simulink model "OMAP"  (R2018b)
settings: Solver=FixedStepDiscrete  StartTime=0.0  StopTime=10.0  FixedStep=0.01  RelTol=1e-3
values from neighbouring files (symbols this model uses):
  Clb_ICADirect_LaneDisp_StateFive = Simulink.Parameter    [omap_ver_442.m]
  Clb_ICADirect_LaneDisp_StateFour = Simulink.Parameter    [omap_ver_442.m]
  Clb_ICADirect_LaneDisp_StateOne = Simulink.Parameter    [omap_ver_442.m]
  Clb_ICADirect_LaneDisp_StateThree = Simulink.Parameter    [omap_ver_442.m]
  Clb_ICADirect_LaneDisp_StateTwo = Simulink.Parameter    [omap_ver_442.m]
  Clb_ICADirect_LaneDisp_StateZero = Simulink.Parameter    [omap_ver_442.m]
  Clb_ICADirect_LaneDispSW = Simulink.Parameter    [omap_ver_442.m]
  Clb_ICADirect_TrnLghtsCom_Switch = Simulink.Parameter    [omap_ver_442.m]
  Clb_ICADirect_TrnLghtsCom_Value = Simulink.Parameter    [omap_ver_442.m]
  Clb_ICADirect_TrnLghtsCrtl_Inhb = Simulink.Parameter    [omap_ver_442.m]
  OMAP_ACCAEB_EMSESC_Decel = Simulink.Parameter    [omap_ver_442.m]
  OMAP_ACCFCW_IC_Decel = Simulink.Parameter    [omap_ver_442.m]
  OMAP_clb_ACC_RVVReqType = Simulink.Parameter    [omap_ver_442.m]
  OMAP_clb_ACC_RVVReqType_Switch = Simulink.Parameter    [omap_ver_442.m]
  OMAP_clb_ACCHeadwayDisplay = Simulink.Parameter    [omap_ver_442.m]
  OMAP_clb_ACCHeadwayDisplay_Switch = Simulink.Parameter    [omap_ver_442.m]
  OMAP_clb_ACCHeadwayIcon = Simulink.Parameter    [omap_ver_442.m]
  OMAP_clb_ACCHeadwayIcon_Switch = Simulink.Parameter    [omap_ver_442.m]
  OMAP_clb_ACCMessagePrompt = Simulink.Parameter    [omap_ver_442.m]
  OMAP_clb_ACCMessagePrompt_Switch = Simulink.Parameter    [omap_ver_442.m]
  OMAP_clb_ACCRequestEPB = Simulink.Parameter    [omap_ver_442.m]
  OMAP_clb_ACCRequestEPB_Switch = Simulink.Parameter    [omap_ver_442.m]
  OMAP_clb_ACCSetSpeed = Simulink.Parameter    [omap_ver_442.m]
  OMAP_clb_ACCSetSpeed_Switch = Simulink.Parameter    [omap_ver_442.m]
  OMAP_clb_ACCSetSpeedDis = Simulink.Parameter    [omap_ver_442.m]
  OMAP_clb_ACCSetSpeedDis_Switch = Simulink.Parameter    [omap_ver_442.m]
  OMAP_clb_ACCState = Simulink.Parameter    [omap_ver_442.m]
  OMAP_clb_ACCState_Switch = Simulink.Parameter    [omap_ver_442.m]
  OMAP_clb_ACCStatusIconDis = Simulink.Parameter    [omap_ver_442.m]
  OMAP_clb_ACCStatusIconDis_Switch = Simulink.Parameter    [omap_ver_442.m]
  OMAP_clb_ACCTorqueReq = Simulink.Parameter    [omap_ver_442.m]
  OMAP_clb_ACCTorqueReq_Switch = Simulink.Parameter    [omap_ver_442.m]
  OMAP_clb_ADAS_State = Simulink.Parameter    [omap_ver_442.m]
  OMAP_clb_ADAS_State_Switch = Simulink.Parameter    [omap_ver_442.m]
  OMAP_clb_AEBAlertReq = Simulink.Parameter    [omap_ver_442.m]
  OMAP_clb_AEBAlertReq_Switch = Simulink.Parameter    [omap_ver_442.m]
  OMAP_clb_AEBBrakingProg = Simulink.Parameter    [omap_ver_442.m]
  OMAP_clb_AEBBrakingProg_Switch = Simulink.Parameter    [omap_ver_442.m]
  OMAP_clb_AEBFaultStatus = Simulink.Parameter    [omap_ver_442.m]
  OMAP_clb_AEBFaultStatus_Switch = Simulink.Parameter    [omap_ver_442.m]
  OMAP_clb_AEBMassageDisp = Simulink.Parameter    [omap_ver_442.m]
  OMAP_clb_AEBMassageDisp_Switch = Simulink.Parameter    [omap_ver_442.m]
  OMAP_clb_AEBState = Simulink.Parameter    [omap_ver_442.m]
  OMAP_clb_AEBState_Switch = Simulink.Parameter    [omap_ver_442.m]
  OMAP_clb_AEBSwitchStatus = Simulink.Parameter    [omap_ver_442.m]
  OMAP_clb_AEBSwitchStatus_Switch = Simulink.Parameter    [omap_ver_442.m]
  OMAP_clb_BrakeRequest = Simulink.Parameter    [omap_ver_442.m]
  OMAP_clb_BrakeRequest_Switch = Simulink.Parameter    [omap_ver_442.m]
  OMAP_clb_DecelerationSet = Simulink.Parameter    [omap_ver_442.m]
  OMAP_clb_DecelerationSet_Switch = Simulink.Parameter    [omap_ver_442.m]
  OMAP_clb_DecelerationType = Simulink.Parameter    [omap_ver_442.m]
  OMAP_clb_DecelerationType_Switch = Simulink.Parameter    [omap_ver_442.m]
  OMAP_clb_DeclControlReq = Simulink.Parameter    [omap_ver_442.m]
  OMAP_clb_DeclControlReq_Switch = Simulink.Parameter    [omap_ver_442.m]
  OMAP_clb_DownorUpGearMinTime = Simulink.Parameter    [omap_ver_442.m]
  OMAP_clb_DownorUpGearMinTime_Switch = Simulink.Parameter    [omap_ver_442.m]
  OMAP_clb_ELKPopupMessage = Simulink.Parameter    [omap_ver_442.m]
  OMAP_clb_ELKPopupMessage_Switch = Simulink.Parameter    [omap_ver_442.m]
  OMAP_clb_ELKSts = Simulink.Parameter    [omap_ver_442.m]
  OMAP_clb_ELKSts_Switch = Simulink.Parameter    [omap_ver_442.m]
  OMAP_clb_ESAFaultSt = Simulink.Parameter    [omap_ver_442.m]
  OMAP_clb_ESAFaultSt_Switch = Simulink.Parameter    [omap_ver_442.m]
  OMAP_clb_ESARequest = Simulink.Parameter    [omap_ver_442.m]
  OMAP_clb_ESARequest_Switch = Simulink.Parameter    [omap_ver_442.m]
  OMAP_clb_ESAState = Simulink.Parameter    [omap_ver_442.m]
  OMAP_clb_ESAState_Switch = Simulink.Parameter    [omap_ver_442.m]
  OMAP_clb_ESATorqueReq = Simulink.Parameter    [omap_ver_442.m]
  OMAP_clb_ESATorqueReq_Switch = Simulink.Parameter    [omap_ver_442.m]
  OMAP_clb_ESCDriveOff = Simulink.Parameter    [omap_ver_442.m]
  OMAP_clb_ESCDriveOff_Switch = Simulink.Parameter    [omap_ver_442.m]
  OMAP_clb_ESCHoldReq = Simulink.Parameter    [omap_ver_442.m]
  OMAP_clb_ESCHoldReq_Switch = Simulink.Parameter    [omap_ver_442.m]
  OMAP_clb_Handsoffwarning = Simulink.Parameter    [omap_ver_442.m]
  OMAP_clb_Handsoffwarning_Switch = Simulink.Parameter    [omap_ver_442.m]
  OMAP_clb_HapticAlarmReq = Simulink.Parameter    [omap_ver_442.m]
  OMAP_clb_HapticAlarmReq_Switch = Simulink.Parameter    [omap_ver_442.m]
  OMAP_clb_HMIPopupMassage = Simulink.Parameter    [omap_ver_442.m]
  OMAP_clb_HMIPopupMassage_Switch = Simulink.Parameter    [omap_ver_442.m]
  OMAP_clb_HWAActionSts = Simulink.Parameter    [omap_ver_442.m]
  OMAP_clb_HWAActionSts_Switch = Simulink.Parameter    [omap_ver_442.m]
  OMAP_clb_HWAMode = Simulink.Parameter    [omap_ver_442.m]
  OMAP_clb_HWAMode_Switch = Simulink.Parameter    [omap_ver_442.m]
  OMAP_clb_HWATurnOnIdctr = Simulink.Parameter    [omap_ver_442.m]
  OMAP_clb_HWATurnOnIdctr_Switch = Simulink.Parameter    [omap_ver_442.m]
  OMAP_clb_ICAMassageDisp = Simulink.Parameter    [omap_ver_442.m]
  OMAP_clb_ICAMassageDisp_Switch = Simulink.Parameter    [omap_ver_442.m]
  OMAP_clb_ICAStatusIcon = Simulink.Parameter    [omap_ver_442.m]
  OMAP_clb_ICAStatusIcon_Switch = Simulink.Parameter    [omap_ver_442.m]
  OMAP_clb_ISLCDriverRemind = Simulink.Parameter    [omap_ver_442.m]
  OMAP_clb_ISLCDriverRemind_Switch = Simulink.Parameter    [omap_ver_442.m]
  OMAP_clb_ISLCState = Simulink.Parameter    [omap_ver_442.m]
  OMAP_clb_ISLCState_Switch = Simulink.Parameter    [omap_ver_442.m]
  OMAP_clb_JAFaultSt = Simulink.Parameter    [omap_ver_442.m]
  OMAP_clb_JAFaultSt_Switch = Simulink.Parameter    [omap_ver_442.m]
  OMAP_clb_LCAPopupMessage = Simulink.Parameter    [omap_ver_442.m]
  OMAP_clb_LCAPopupMessage_Switch = Simulink.Parameter    [omap_ver_442.m]
  OMAP_clb_LCAStatusDisplay = Simulink.Parameter    [omap_ver_442.m]
  OMAP_clb_LCAStatusDisplay_Switch = Simulink.Parameter    [omap_ver_442.m]
  OMAP_clb_LDWStatusDisplay = Simulink.Parameter    [omap_ver_442.m]
  OMAP_clb_LDWStatusDisplay_Switch = Simulink.Parameter    [omap_ver_442.m]
  OMAP_clb_LDWWarningSt = Simulink.Parameter    [omap_ver_442.m]
  OMAP_clb_LDWWarningSt_Switch = Simulink.Parameter    [omap_ver_442.m]
  OMAP_clb_LightControlValid = Simulink.Parameter    [omap_ver_442.m]
  OMAP_clb_LightControlValid_Switch = Simulink.Parameter    [omap_ver_442.m]
  OMAP_clb_LKAActivation = Simulink.Parameter    [omap_ver_442.m]
  OMAP_clb_LKAActivation_Switch = Simulink.Parameter    [omap_ver_442.m]
  OMAP_clb_LKAAngleReq = Simulink.Parameter    [omap_ver_442.m]
  OMAP_clb_LKAAngleReq_Switch = Simulink.Parameter    [omap_ver_442.m]
  OMAP_clb_LKAMode = Simulink.Parameter    [omap_ver_442.m]
  OMAP_clb_LKAMode_Switch = Simulink.Parameter    [omap_ver_442.m]
  OMAP_clb_LKAorELK_CoolTime = Simulink.Parameter    [omap_ver_442.m]
  OMAP_clb_LKAState = Simulink.Parameter    [omap_ver_442.m]
  OMAP_clb_LKAState_Switch = Simulink.Parameter    [omap_ver_442.m]
  OMAP_clb_LKAStatusDisplay = Simulink.Parameter    [omap_ver_442.m]
  OMAP_clb_LKAStatusDisplay_Switch = Simulink.Parameter    [omap_ver_442.m]
  OMAP_clb_LKASwitchState = Simulink.Parameter    [omap_ver_442.m]
  OMAP_clb_LKASwitchState_Switch = Simulink.Parameter    [omap_ver_442.m]
  OMAP_clb_LKATorqFactReq = Simulink.Parameter    [omap_ver_442.m]
  OMAP_clb_LKATorqFactReq_Switch = Simulink.Parameter    [omap_ver_442.m]
  OMAP_clb_PrefillRequest = Simulink.Parameter    [omap_ver_442.m]
  ... (+36 more)
libraries: simulink x184, canmsglib x2
(part 7 of 14)

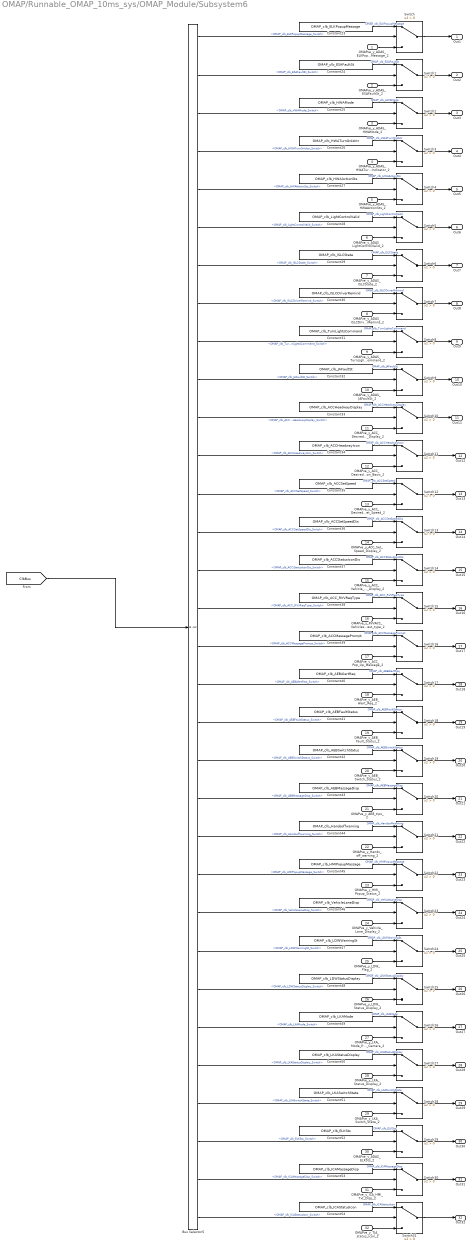
== system OMAP/Runnable_OMAP_10ms_sys/OMAP_Module/Subsystem6 ==
  OMAPve_y_ADAS_ELKPopupMessage_2 : Inport
  OMAPve_y_ADAS_ESAFaultSt_2 : Inport  Port=2
  OMAPve_y_ADAS_HWAMode_2 : Inport  Port=3
  OMAPve_y_ADAS_HWATurnOnIndicator_2 : Inport  Port=4
  OMAPve_y_ADAS_HWAActionSts_2 : Inport  Port=5
  OMAPve_y_ADAS_LightControlValid_2 : Inport  Port=6
  OMAPve_y_ADAS_ISLCState_2 : Inport  Port=7
  OMAPve_y_ADAS_ISLCDriverRemind_2 : Inport  Port=8
  OMAPve_y_ADAS_TurnLightsCommand_2 : Inport  Port=9
  OMAPve_y_ADAS_JAFaultSt_2 : Inport  Port=10
  OMAPve_y_ACC_DesiredHeadway_Display_2 : Inport  Port=11
  OMAPve_y_ACC_DesiredHeadway_Icon_Basic_2 : Inport  Port=12
  OMAPve_y_ACC_Desired_Set_Speed_2 : Inport  Port=13
  OMAPve_y_ACC_Set_Speed_Display_2 : Inport  Port=14
  OMAPve_y_ACC_Vehicle_Icon_Display_2 : Inport  Port=15
  OMAPve_y_RVVACC_Vehiclespeed_request_type_2 : Inport  Port=16
  OMAPve_y_ACC_Pop_Up_Message_2 : Inport  Port=17
  OMAPve_y_AEB_Alert_Req_2 : Inport  Port=18
  OMAPve_y_AEB_Fault_Status_2 : Inport  Port=19
  OMAPve_y_AEB_Switch_Status_2 : Inport  Port=20
  OMAPve_y_AEB_tips_2 : Inport  Port=21
  OMAPve_y_Hands_off_warning_2 : Inport  Port=22
  OMAPve_y_HMI_Popup_Status_2 : Inport  Port=23
  OMAPve_y_Vehicle_Lane_Display_2 : Inport  Port=24
  OMAPve_y_LDW_Flag_2 : Inport  Port=25
  OMAPve_y_LDW_Status_Display_2 : Inport  Port=26
  OMAPve_y_LKA_Mode_from_Camera_2 : Inport  Port=27
  OMAPve_y_LKA_Status_Display_2 : Inport  Port=28
  OMAPve_y_LKA_Switch_State_2 : Inport  Port=29
  OMAPve_y_ADAS_ELKSts_2 : Inport  Port=30
  OMAPve_y_ICA_HMI_Txt_Disp_2 : Inport  Port=31
  OMAPve_y_TJA_status_icon_2 : Inport  Port=32
  Bus Selector5 : BusSelector  OutputSignals=OMAP_clb_ELKPopupMessage_Switch,OMAP_clb_ESAFaultSt_Switch,OMAP_clb_HWAMode_Switch,OMAP_clb_HWATurnOnIdctr_Switch,OMAP_clb_HWAActionSts_Switch,OMAP_clb_LightControlValid_Switch,OMAP_clb_ISLCState_Switch,OMAP_clb_ISLCDriverRemind_Switch,OMAP_clb_TurnLightsCommand_Switch,OMAP_clb_JAFaultSt_Switch,OMAP_clb_ACCHeadwayDisplay_Switch,OMAP_clb_ACCHeadwayIcon_Switch,OMAP_clb_ACCSetSpeed_Switch,OMAP_clb_ACCSetSpeedDis_Switch,OMAP_clb_ACCStatusIconDis_Switch,OMAP_clb_ACC_RVVReqType_Switch,OMAP_clb_ACCMessagePrompt_Switch,OMAP_clb_AEBAlertReq_Switch,OMAP_clb_AEBFaultStatus_Switch,OMAP_clb_AEBSwitchStatus_Switch,OMAP_clb_AEBMassageDisp_Switch,OMAP_clb_Handsoffwarning_Switch,OMAP_clb_HMIPopupMassage_Switch,OMAP_clb_VehicleLaneDisp_Switch,OMAP_clb_LDWWarningSt_Switch,OMAP_clb_LDWStatusDisplay_Switch,OMAP_clb_LKAMode_Switch,OMAP_clb_LKAStatusDisplay_Switch,OMAP_clb_LKASwitchState_Switch,OMAP_clb_ELKSts_Switch,OMAP_clb_ICAMassageDisp_Switch,OMAP_clb_ICAStatusIcon_Switch
  Constant23 : Constant  Value=OMAP_clb_ELKPopupMessage
  Constant24 : Constant  Value=OMAP_clb_ESAFaultSt
  Constant25 : Constant  Value=OMAP_clb_HWAMode
  Constant26 : Constant  Value=OMAP_clb_HWATurnOnIdctr
  Constant27 : Constant  Value=OMAP_clb_HWAActionSts
  Constant28 : Constant  Value=OMAP_clb_LightControlValid
  Constant29 : Constant  Value=OMAP_clb_ISLCState
  Constant30 : Constant  Value=OMAP_clb_ISLCDriverRemind
  Constant31 : Constant  Value=OMAP_clb_TurnLightsCommand
  Constant32 : Constant  Value=OMAP_clb_JAFaultSt
  Constant33 : Constant  Value=OMAP_clb_ACCHeadwayDisplay
  Constant34 : Constant  Value=OMAP_clb_ACCHeadwayIcon
  Constant35 : Constant  Value=OMAP_clb_ACCSetSpeed
  Constant36 : Constant  Value=OMAP_clb_ACCSetSpeedDis
  Constant37 : Constant  Value=OMAP_clb_ACCStatusIconDis
  Constant38 : Constant  Value=OMAP_clb_ACC_RVVReqType
  Constant39 : Constant  Value=OMAP_clb_ACCMessagePrompt
  Constant40 : Constant  Value=OMAP_clb_AEBAlertReq
  Constant41 : Constant  Value=OMAP_clb_AEBFaultStatus
  Constant42 : Constant  Value=OMAP_clb_AEBSwitchStatus
  Constant43 : Constant  Value=OMAP_clb_AEBMassageDisp
  Constant44 : Constant  Value=OMAP_clb_Handsoffwarning
  Constant45 : Constant  Value=OMAP_clb_HMIPopupMassage
  Constant46 : Constant  Value=OMAP_clb_VehicleLaneDisp
  Constant47 : Constant  Value=OMAP_clb_LDWWarningSt
  Constant48 : Constant  Value=OMAP_clb_LDWStatusDisplay
  Constant49 : Constant  Value=OMAP_clb_LKAMode
  Constant50 : Constant  Value=OMAP_clb_LKAStatusDisplay
  Constant51 : Constant  Value=OMAP_clb_LKASwitchState
  Constant52 : Constant  Value=OMAP_clb_ELKSts
  Constant53 : Constant  Value=OMAP_clb_ICAMassageDisp
  Constant54 : Constant  Value=OMAP_clb_ICAStatusIcon
  Switch{,1..31} (32 alike) : Switch  Criteria=u2 > Threshold
  Out1 : Outport
  Out2 : Outport  Port=2
  Out3 : Outport  Port=3
  Out4 : Outport  Port=4
  Out5 : Outport  Port=5
  Out6 : Outport  Port=6
  Out7 : Outport  Port=7
  Out8 : Outport  Port=8
  Out9 : Outport  Port=9
  Out10 : Outport  Port=10
  Out11 : Outport  Port=11
  Out12 : Outport  Port=12
  Out13 : Outport  Port=13
  Out14 : Outport  Port=14
  Out15 : Outport  Port=15
  Out16 : Outport  Port=16
  Out17 : Outport  Port=17
  Out18 : Outport  Port=18
  Out19 : Outport  Port=19
  Out20 : Outport  Port=20
  Out21 : Outport  Port=21
  Out22 : Outport  Port=22
  Out23 : Outport  Port=23
  Out24 : Outport  Port=24
  Out25 : Outport  Port=25
  Out26 : Outport  Port=26
  Out27 : Outport  Port=27
  Out28 : Outport  Port=28
  Out29 : Outport  Port=29
  Out30 : Outport  Port=30
  Out31 : Outport  Port=31
  Out32 : Outport  Port=32
  wires:
  Switch10/1 -> Out11/1
  OMAPve_y_ACC_DesiredHeadway_Display_2/1 -> Switch10/3
  Bus Selector5/11 -> Switch10/2  "<OMAP_clb_ACCHeadwayDisplay_Switch>"
  OMAPve_y_ADAS_JAFaultSt_2/1 -> Switch9/3
  Switch9/1 -> Out10/1
  Bus Selector5/10 -> Switch9/2  "<OMAP_clb_JAFaultSt_Switch>"
  OMAPve_y_ADAS_TurnLightsCommand_2/1 -> Switch8/3
  Bus Selector5/9 -> Switch8/2  "<OMAP_clb_TurnLightsCommand_Switch>"
  Switch8/1 -> Out9/1
  Switch7/1 -> Out8/1
  OMAPve_y_ADAS_ISLCDriverRemind_2/1 -> Switch7/3
  Bus Selector5/8 -> Switch7/2  "<OMAP_clb_ISLCDriverRemind_Switch>"
  Switch6/1 -> Out7/1
  OMAPve_y_ADAS_ISLCState_2/1 -> Switch6/3
  Bus Selector5/7 -> Switch6/2  "<OMAP_clb_ISLCState_Switch>"
  Switch5/1 -> Out6/1
  OMAPve_y_ADAS_LightControlValid_2/1 -> Switch5/3
  Bus Selector5/6 -> Switch5/2  "<OMAP_clb_LightControlValid_Switch>"
  Switch4/1 -> Out5/1
  Bus Selector5/5 -> Switch4/2  "<OMAP_clb_HWAActionSts_Switch>"
  OMAPve_y_ADAS_HWAActionSts_2/1 -> Switch4/3
  Bus Selector5/2 -> Switch1/2  "<OMAP_clb_ESAFaultSt_Switch>"
  Switch2/1 -> Out3/1
  OMAPve_y_ADAS_HWATurnOnIndicator_2/1 -> Switch3/3
  OMAPve_y_ADAS_HWAMode_2/1 -> Switch2/3
  OMAPve_y_ADAS_ESAFaultSt_2/1 -> Switch1/3
  Bus Selector5/1 -> Switch/2  "<OMAP_clb_ELKPopupMessage_Switch>"
  [ClbBus] -> Bus Selector5/1
  Bus Selector5/3 -> Switch2/2  "<OMAP_clb_HWAMode_Switch>"
  Bus Selector5/4 -> Switch3/2  "<OMAP_clb_HWATurnOnIdctr_Switch>"
  OMAPve_y_ADAS_ELKPopupMessage_2/1 -> Switch/3
  Switch1/1 -> Out2/1
  Switch3/1 -> Out4/1
  Switch/1 -> Out1/1
  Bus Selector5/12 -> Switch11/2  "<OMAP_clb_ACCHeadwayIcon_Switch>"
  OMAPve_y_ACC_DesiredHeadway_Icon_Basic_2/1 -> Switch11/3
  Switch11/1 -> Out12/1
  Bus Selector5/13 -> Switch12/2  "<OMAP_clb_ACCSetSpeed_Switch>"
  OMAPve_y_ACC_Desired_Set_Speed_2/1 -> Switch12/3
  Switch12/1 -> Out13/1
  Switch13/1 -> Out14/1
  OMAPve_y_ACC_Set_Speed_Display_2/1 -> Switch13/3
  Bus Selector5/14 -> Switch13/2  "<OMAP_clb_ACCSetSpeedDis_Switch>"
  Bus Selector5/15 -> Switch14/2  "<OMAP_clb_ACCStatusIconDis_Switch>"
  OMAPve_y_ACC_Vehicle_Icon_Display_2/1 -> Switch14/3
  Switch14/1 -> Out15/1
  Switch15/1 -> Out16/1
  OMAPve_y_RVVACC_Vehiclespeed_request_type_2/1 -> Switch15/3
  Bus Selector5/16 -> Switch15/2  "<OMAP_clb_ACC_RVVReqType_Switch>"
  Bus Selector5/17 -> Switch16/2  "<OMAP_clb_ACCMessagePrompt_Switch>"
  OMAPve_y_ACC_Pop_Up_Message_2/1 -> Switch16/3
  Switch16/1 -> Out17/1
  Switch17/1 -> Out18/1
  OMAPve_y_AEB_Alert_Req_2/1 -> Switch17/3
  Bus Selector5/18 -> Switch17/2  "<OMAP_clb_AEBAlertReq_Switch>"
  Bus Selector5/19 -> Switch18/2  "<OMAP_clb_AEBFaultStatus_Switch>"
  OMAPve_y_AEB_Fault_Status_2/1 -> Switch18/3
  Switch18/1 -> Out19/1
  Switch19/1 -> Out20/1
  OMAPve_y_AEB_Switch_Status_2/1 -> Switch19/3
  Bus Selector5/20 -> Switch19/2  "<OMAP_clb_AEBSwitchStatus_Switch>"
  Bus Selector5/21 -> Switch20/2  "<OMAP_clb_AEBMassageDisp_Switch>"
  OMAPve_y_AEB_tips_2/1 -> Switch20/3
  Switch20/1 -> Out21/1
  Switch21/1 -> Out22/1
  OMAPve_y_Hands_off_warning_2/1 -> Switch21/3
  Bus Selector5/22 -> Switch21/2  "<OMAP_clb_Handsoffwarning_Switch>"
  Bus Selector5/23 -> Switch22/2  "<OMAP_clb_HMIPopupMassage_Switch>"
  OMAPve_y_HMI_Popup_Status_2/1 -> Switch22/3
  Switch22/1 -> Out23/1
  Switch23/1 -> Out24/1
  OMAPve_y_Vehicle_Lane_Display_2/1 -> Switch23/3
  Bus Selector5/24 -> Switch23/2  "<OMAP_clb_VehicleLaneDisp_Switch>"
  Bus Selector5/25 -> Switch24/2  "<OMAP_clb_LDWWarningSt_Switch>"
  OMAPve_y_LDW_Flag_2/1 -> Switch24/3
  Switch24/1 -> Out25/1
  Switch25/1 -> Out26/1
  OMAPve_y_LDW_Status_Display_2/1 -> Switch25/3
  Bus Selector5/26 -> Switch25/2  "<OMAP_clb_LDWStatusDisplay_Switch>"
  Bus Selector5/27 -> Switch26/2  "<OMAP_clb_LKAMode_Switch>"
  OMAPve_y_LKA_Mode_from_Camera_2/1 -> Switch26/3
  Switch26/1 -> Out27/1
  Switch27/1 -> Out28/1
  OMAPve_y_LKA_Status_Display_2/1 -> Switch27/3
  Bus Selector5/28 -> Switch27/2  "<OMAP_clb_LKAStatusDisplay_Switch>"
  Bus Selector5/29 -> Switch28/2  "<OMAP_clb_LKASwitchState_Switch>"
  OMAPve_y_LKA_Switch_State_2/1 -> Switch28/3
  Switch28/1 -> Out29/1
  Switch29/1 -> Out30/1
  OMAPve_y_ADAS_ELKSts_2/1 -> Switch29/3
  Bus Selector5/30 -> Switch29/2  "<OMAP_clb_ELKSts_Switch>"
  Bus Selector5/31 -> Switch30/2  "<OMAP_clb_ICAMassageDisp_Switch>"
  OMAPve_y_ICA_HMI_Txt_Disp_2/1 -> Switch30/3
  Switch30/1 -> Out31/1
  Switch31/1 -> Out32/1
  OMAPve_y_TJA_status_icon_2/1 -> Switch31/3
  Bus Selector5/32 -> Switch31/2  "<OMAP_clb_ICAStatusIcon_Switch>"
  Constant23/1 -> Switch/1  "OMAP_clb_ELKPopupMessage"
  Constant24/1 -> Switch1/1  "OMAP_clb_ESAFaultSt"
  Constant25/1 -> Switch2/1  "OMAP_clb_HWAMode"
  Constant26/1 -> Switch3/1  "OMAP_clb_HWATurnOnIdctr"
  Constant27/1 -> Switch4/1  "OMAP_clb_HWAActionSts"
  Constant28/1 -> Switch5/1  "OMAP_clb_LightControlValid"
  Constant29/1 -> Switch6/1  "OMAP_clb_ISLCState"
  Constant30/1 -> Switch7/1  "OMAP_clb_ISLCDriverRemind"
  Constant31/1 -> Switch8/1  "OMAP_clb_TurnLightsCommand"
  Constant32/1 -> Switch9/1  "OMAP_clb_JAFaultSt"
  Constant33/1 -> Switch10/1  "OMAP_clb_ACCHeadwayDisplay"
  Constant34/1 -> Switch11/1  "OMAP_clb_ACCHeadwayIcon"
  Constant35/1 -> Switch12/1  "OMAP_clb_ACCSetSpeed"
  Constant36/1 -> Switch13/1  "OMAP_clb_ACCSetSpeedDis"
  Constant37/1 -> Switch14/1  "OMAP_clb_ACCStatusIconDis"
  Constant38/1 -> Switch15/1  "OMAP_clb_ACC_RVVReqType"
  Constant39/1 -> Switch16/1  "OMAP_clb_ACCMessagePrompt"
  Constant40/1 -> Switch17/1  "OMAP_clb_AEBAlertReq"
  Constant41/1 -> Switch18/1  "OMAP_clb_AEBFaultStatus"
  Constant42/1 -> Switch19/1  "OMAP_clb_AEBSwitchStatus"
  Constant43/1 -> Switch20/1  "OMAP_clb_AEBMassageDisp"
  Constant44/1 -> Switch21/1  "OMAP_clb_Handsoffwarning"
  Constant45/1 -> Switch22/1  "OMAP_clb_HMIPopupMassage"
  Constant46/1 -> Switch23/1  "OMAP_clb_VehicleLaneDisp"
  Constant47/1 -> Switch24/1  "OMAP_clb_LDWWarningSt"
  Constant48/1 -> Switch25/1  "OMAP_clb_LDWStatusDisplay"
  Constant49/1 -> Switch26/1  "OMAP_clb_LKAMode"
  Constant50/1 -> Switch27/1  "OMAP_clb_LKAStatusDisplay"
  Constant51/1 -> Switch28/1  "OMAP_clb_LKASwitchState"
  Constant52/1 -> Switch29/1  "OMAP_clb_ELKSts"
  Constant53/1 -> Switch30/1  "OMAP_clb_ICAMassageDisp"
  Constant54/1 -> Switch31/1  "OMAP_clb_ICAStatusIcon"

== system OMAP/Runnable_OMAP_10ms_sys/OMAP_Module/Subsystem7 ==
  OMAPve_y_ADAS_LCAStatusDisplay1 : Inport
  OMAPve_y_ADAS_LCAPopupMessage1 : Inport  Port=2
  OMAPve_y_ADAS_State1 : Inport  Port=3
  Bus Selector5 : BusSelector  OutputSignals=OMAP_clb_LCAStatusDisplay_Switch,OMAP_clb_LCAPopupMessage_Switch,OMAP_clb_ADAS_State_Switch
  Constant55 : Constant  Value=OMAP_clb_LCAStatusDisplay
  Constant56 : Constant  Value=OMAP_clb_LCAPopupMessage
  Constant57 : Constant  Value=OMAP_clb_ADAS_State
  Switch : Switch  Criteria=u2 > Threshold
  Switch1 : Switch  Criteria=u2 > Threshold
  Switch2 : Switch  Criteria=u2 > Threshold
  Out1 : Outport
  Out2 : Outport  Port=2
  Out3 : Outport  Port=3
  wires:
  Switch/1 -> Out1/1
  Switch1/1 -> Out2/1
  OMAPve_y_ADAS_LCAStatusDisplay1/1 -> Switch/3
  Bus Selector5/3 -> Switch2/2  "<OMAP_clb_ADAS_State_Switch>"
  [ClbBus] -> Bus Selector5/1
  Bus Selector5/1 -> Switch/2  "<OMAP_clb_LCAStatusDisplay_Switch>"
  OMAPve_y_ADAS_LCAPopupMessage1/1 -> Switch1/3
  OMAPve_y_ADAS_State1/1 -> Switch2/3
  Switch2/1 -> Out3/1
  Bus Selector5/2 -> Switch1/2  "<OMAP_clb_LCAPopupMessage_Switch>"
  Constant55/1 -> Switch/1  "OMAP_clb_LCAStatusDisplay"
  Constant56/1 -> Switch1/1  "OMAP_clb_LCAPopupMessage"
  Constant57/1 -> Switch2/1  "OMAP_clb_ADAS_State"

== system OMAP/Runnable_OMAP_10ms_sys/OMAP_Module/Subsystem8 ==
  OMAPve_y_TYPE_RAPPORT_2 : Inport
  Bus Selector5 : BusSelector  OutputSignals=OMAP_clb_UpDownGearChange_Switch
  Constant22 : Constant  Value=OMAP_clb_UpDownGearChange
  Switch : Switch  Criteria=u2 > Threshold
  Out1 : Outport
  wires:
  Bus Selector5/1 -> Switch/2  "<OMAP_clb_UpDownGearChange_Switch>"
  [ClbBus] -> Bus Selector5/1
  OMAPve_y_TYPE_RAPPORT_2/1 -> Switch/3
  Switch/1 -> Out1/1
  Constant22/1 -> Switch/1  "OMAP_clb_UpDownGearChange"

== system OMAP/Runnable_OMAP_10ms_sys/OMAP_Module/ACCS_Direct/ACCS_Define ==
  In1 : Inport
  In2 : Inport  Port=2
  In3 : Inport  Port=3
  ACC_State_Synthesis(ACC_SS) : Subsystem
  Bus Creator : BusCreator  Inputs=13
  Bus Selector1 : BusSelector  OutputSignals=ACCSve_d_CIPV_ID_convert,ACCSve_d_ACC_State_convert,ACCSve_d_ACCActive_Signal_convert,ACCSve_d_ACC_ICA_Flag_convert,ACCSve_d_HeadWaySet_convert,ACCSve_d_VelocitySet_convert,ACCSve_d_ACC_go_request_convert,ACCSve_g_ACC_DecReq_convert,ACCSve_d_ACC_ISLCState_convert,ACCSve_d_ACC_ISLCDriverRemind_convert,ACCSve_d_ACCMessagePrompt_convert
  Bus Selector2 : BusSelector  OutputSignals=IMAPva_d_obj_id_convert,IMAPva_g_obj_pos_x_convert
  CIPV_Data : MATLAB Function  TreatAsAtomicUnit=on
  Human_Machine_Interface(ACC_HMI) : Subsystem
  Terminator1 : Terminator
  Out1 : Outport
  Out2 : Outport  Port=2
  tag scope: CIPV_ID=global, CIPV_ID_Longitudinal_Distance=global
  wires:
  ACC_State_Synthesis(ACC_SS)/1(ACC_Control_Signal) -> Out1/1
  In2/1 -> Terminator1/1
  In1/1 -> Bus Selector1/1, ACC_State_Synthesis(ACC_SS)/1(Input_ACCS)
  Human_Machine_Interface(ACC_HMI)/1(ACC_DesiredHeadway_Display) -> Bus Creator/1  "OMAPve_y_ACC_DesiredHeadway_Display_2"
  Human_Machine_Interface(ACC_HMI)/2(ACC_DesiredHeadway_Icon_Basic) -> Bus Creator/2  "OMAPve_y_ACC_DesiredHeadway_Icon_Basic_2"
  Human_Machine_Interface(ACC_HMI)/3(ACC_Desired_Set_Speed) -> Bus Creator/3  "OMAPve_y_ACC_Desired_Set_Speed_2"
  Human_Machine_Interface(ACC_HMI)/4(ACC_Set_Speed_Display) -> Bus Creator/4  "OMAPve_y_ACC_Set_Speed_Display_2"
  Human_Machine_Interface(ACC_HMI)/5(ACC_Vehicle_Icon_Display) -> Bus Creator/5  "OMAPve_y_ACC_Vehicle_Icon_Display_2"
  Human_Machine_Interface(ACC_HMI)/6(RVVACC_Vehiclespeed_request_type) -> Bus Creator/6  "OMAPve_y_RVVACC_Vehiclespeed_request_type_2"
  Bus Selector1/10 -> Bus Creator/13  "<ACCSve_d_ACC_ISLCDriverRemind_convert>"
  Human_Machine_Interface(ACC_HMI)/8(ACC_HMI_TgDisp_Flag) -> Bus Creator/8  "OMAPve_y_ACC_HMI_TgtDisp_Flag_2"
  Human_Machine_Interface(ACC_HMI)/9(TARGET_POSITION) -> Bus Creator/9  "OMAPve_y_TARGET_POSITION_2"
  Human_Machine_Interface(ACC_HMI)/10(ACC_Pop_Up_Message_TJA) -> Bus Creator/10  "ACC_Pop_Up_Message_TJA"
  Bus Creator/1 -> Out2/1
  Bus Selector1/7 -> Human_Machine_Interface(ACC_HMI)/8(ACC_go_request)  "<ACCSve_d_ACC_go_request_convert>"
  Bus Selector1/4 -> Human_Machine_Interface(ACC_HMI)/5(ACC_ICA_Flag)  "<ACCSve_d_ACC_ICA_Flag_convert>"
  Bus Selector1/1 -> CIPV_Data/3(ACCSve_d_CIPV_ID), [CIPV_ID], Human_Machine_Interface(ACC_HMI)/2(CIPV_ID)  "<ACCSve_d_CIPV_ID_convert>"
  Bus Selector1/5 -> Human_Machine_Interface(ACC_HMI)/6(HeadWaySet)  "<ACCSve_d_HeadWaySet_convert>"
  CIPV_Data/1(CIPV_ID_Longitudinal_Distance) -> [CIPV_ID_Longitudinal_Distance], Human_Machine_Interface(ACC_HMI)/1(CIPV_ID_Longitudinal_Distance)
  Bus Selector1/3 -> Human_Machine_Interface(ACC_HMI)/4(ACCActive_Signal)  "<ACCSve_d_ACCActive_Signal_convert>"
  Bus Selector1/2 -> Bus Creator/11, Human_Machine_Interface(ACC_HMI)/3(ACC_State)  "<ACCSve_d_ACC_State_convert>"
  Bus Selector1/8 -> Human_Machine_Interface(ACC_HMI)/9(ACC_DecReq)  "<ACCSve_g_ACC_DecReq_convert>"
  Bus Selector2/1 -> CIPV_Data/1(IMAPva_d_obj_id)  "<IMAPva_d_obj_id_convert>"
  Bus Selector2/2 -> CIPV_Data/2(IMAPva_g_obj_pos_x)  "<IMAPva_g_obj_pos_x_convert>"
  Bus Selector1/6 -> Human_Machine_Interface(ACC_HMI)/7(VelocitySet)  "<ACCSve_d_VelocitySet_convert>"
  In3/1 -> Bus Selector2/1
  Bus Selector1/9 -> Bus Creator/12  "<ACCSve_d_ACC_ISLCState_convert>"
  Bus Selector1/11 -> Bus Creator/7  "<ACCSve_d_ACCMessagePrompt_convert>"

== system OMAP/Runnable_OMAP_10ms_sys/OMAP_Module/ICA_Direct_G59/ICA_Define ==
  note: 0 ：不可以从降级回到正常，
      | 1 ：可以从降级回到正常
  note: 推荐变道打转向灯
  note: 功能键状态
  note: 有没有方向盘限幅的影响
  note: 为放弃变道的接管提醒预留
  note: 已修改：0是脱手，1是不脱手
  note: 0是静止，1是运动
  note: 推荐变道打转向灯有效性
  note: 转向灯状态
  note: ICA多车道模式开关状态
  note: 0：不亮
      | 1：左转灯亮
      | 2：右转灯亮
      | 3：双闪
  note: 0：无效
      | 1：有效
  note: 能否从降级回到正常
  note: 0 ：变道等待
      | 1 ：向左变道阶段
      | 2：向右变道阶段
  note: LF状态，暂时未用
  note: 0 ：不提醒
      | 1 ：提醒
  note: 变道速度条件满足标志位
  note: 0：速度低于变道门槛值
      | 1：速度高于变道门槛值
  note: FDMM转译后——
      | 0：OFF
      | 1：ICA
      | 2：TLC
      | 3：ALC+TLC
  note: 0 属于CD状态不输出任何Req
      | 1 属于Start状态开始Judge输出L or R
      | 2 Left推荐变道使能
      | 3 Right 推荐变道使能
  In1 : Inport
  In3 : Inport  Port=2
  In2 : Inport  Port=3
  In4 : Inport  Port=4
  Bus Creator : BusCreator  Inputs=7
  Bus Creator1 : BusCreator  Inputs=11
  Bus Selector : BusSelector  OutputSignals=IMAPve_d_EPS_LKA_State_convert,IMAPve_d_ESC_Veh_Standstill_convert,IMAPve_g_L0_C0_convert,IMAPve_g_L0_C1_convert,IMAPve_g_L0_C2_convert,IMAPve_g_L0_C3_convert,IMAPve_g_R0_C0_convert,IMAPve_g_R0_C1_convert,IMAPve_g_R0_C2_convert,IMAPve_g_R0_C3_convert
  Bus Selector11 : BusSelector  OutputSignals=ICABve_d_ICAState_convert,ICABve_g_SteerAngleCmd_convert,ICABve_d_LKATorqueReq_convert,ICABve_g_LKATorqueReq_Value_convert,ICABva_d_ICAB2HMI_convert
  Bus Selector2 : BusSelector  OutputSignals=ACCSve_d_ACC_State_convert,ACC_Pop_Up_Message_TJA
  Demux : Demux  Outputs=20
  ICA_EPS : Subsystem
  Subsystem1 : Subsystem
  TH_HMIClb : Subsystem  Description=|
      | Block Name:TH_VFClb
      | No.: THC.05
      | Rev: 00.00.01
      | Update Date: 19-3-28
  Terminator : Terminator
  Out1 : Outport
  Out2 : Outport  Port=2
  wires:
  In2/1 -> Bus Selector/1
  Bus Selector/1 -> ICA_EPS/5(EPSPCEM_stEPSCtlState)  "<IMAPve_d_EPS_LKA_State_convert>"
  TH_HMIClb/1(Out) -> Subsystem1/32(HMI_Clb)  "TH_HMIClb"
  Subsystem1/6(Hands_off_warning) -> Bus Creator1/6  "OMAPve_y_Hands_off_warning_2"
  Subsystem1/5(ISA_Value) -> Bus Creator1/5  "OMAPve_y_ISA_Value_2"
  Subsystem1/4(Vehiclr_Line_Display) -> Bus Creator1/4  "OMAPve_y_Vehicle_Lane_Display_2"
  Subsystem1/1(Dspl_stTxtDspl) -> Bus Creator1/1  "OMAPve_y_ICA_HMI_Txt_Disp_2"
  Subsystem1/3(TSR_Version_Only_Sign_Type) -> Bus Creator1/3  "OMAPve_y_TSR_Vision_Only_Sign_Type_2"
  Subsystem1/2(Dspl_stICAIcon) -> Bus Creator1/2  "OMAPve_y_TJA_status_icon_2"
  Bus Creator1/1 -> Out2/1
  In3/1 -> Terminator/1
  In4/1 -> Bus Selector2/1
  Demux/1 -> Subsystem1/12(EPSRx_stHandOff)  "[1]stHandOff"
  Demux/2 -> Subsystem1/13(EPSRx_stTkOvStChk)  "[2]stTkOvStChk"
  Demux/3 -> Subsystem1/14(L0QI_Opt)  "[3]facmL0QIDisp"
  Demux/4 -> Subsystem1/15(R0QI_Opt)  "[4]facmR0QIDisp"
  Demux/5 -> Subsystem1/16(L0Type_Opt)  "[5]L0Type_Opt"
  Demux/6 -> Subsystem1/17(R0Type_Opt)  "[6]R0Type_Opt"
  Demux/7 -> Subsystem1/18(stTHState)  "[7]stTHState"
  Demux/8 -> Subsystem1/19(stTHFKeyStt)  "[8]stTHFKeyStt"
  Demux/9 -> Subsystem1/20(stTHAutRydEnaFlg)  "[9]THAutRydEnaFlg"
  Demux/10 -> Subsystem1/21(stSWALimFlg)  "[10]stSWALimFlg"
  Demux/11 -> Subsystem1/22(stTHMode)  "[11]stTHMode"
  Demux/12 -> Subsystem1/23(stLCScene)  "[12]stLCScene"
  Demux/15 -> Subsystem1/26(HMI_tfAddVocCmd)  "[15]tfAddVocCmd"
  Demux/16 -> Subsystem1/27(stLCRMode)  "[16]stLCRmode"
  Bus Selector2/2 -> Subsystem1/11(ACC_HMI_Txt_Disp)  "<ACC_Pop_Up_Message_TJA>"
  Bus Selector2/1 -> Subsystem1/10(ACC_State)  "<ACCSve_d_ACC_State_convert>"
  Bus Selector/2 -> Subsystem1/1(VehMovRx_VehicleStationary)  "<IMAPve_d_ESC_Veh_Standstill_convert>"
  Bus Selector/3 -> Subsystem1/2(L0C0_Org)  "<IMAPve_g_L0_C0_convert>"
  Bus Selector/4 -> Subsystem1/3(L0C1_Org)  "<IMAPve_g_L0_C1_convert>"
  Bus Selector/5 -> Subsystem1/4(L0C2_Org)  "<IMAPve_g_L0_C2_convert>"
  Bus Selector/6 -> Subsystem1/5(L0C3_Org)  "<IMAPve_g_L0_C3_convert>"
  Bus Selector/7 -> Subsystem1/6(R0C0_Org)  "<IMAPve_g_R0_C0_convert>"
  Bus Selector/8 -> Subsystem1/7(R0C1_Org)  "<IMAPve_g_R0_C1_convert>"
  Bus Selector/9 -> Subsystem1/8(R0C2_Org)  "<IMAPve_g_R0_C2_convert>"
  Bus Selector/10 -> Subsystem1/9(R0C3_Org)  "<IMAPve_g_R0_C3_convert>"
  In1/1 -> Bus Selector11/1
  ICA_EPS/5(ICABve_g_SteerAngleCmd_convert) -> Bus Creator/5  "ICABve_g_SteerAngleCmd_convert"
  ICA_EPS/7(ICABve_g_LKATorqueReq_Value_convert) -> Bus Creator/7  "ICABve_g_LKATorqueReq_Value_convert"
  Bus Selector11/5 -> Demux/1  "<ICABva_d_ICAB2HMI_convert>"
  Bus Selector11/1 -> ICA_EPS/1(EPSPCEM_stICAState)  "<ICABve_d_ICAState_convert>"
  Bus Selector11/3 -> ICA_EPS/3(torque_Req)  "<ICABve_d_LKATorqueReq_convert>"
  ICA_EPS/1(stEPS_State_Ctl_CMD) -> Bus Creator/1  "OMAPve_y_General_state_of_LKA_function3F2_2"
  ICA_EPS/3(LKA_OR_LPA_REQ) -> Bus Creator/3  "OMAPve_y_Permit_to_know_if_LKA_or_LPA3F2_2"
  ICA_EPS/4(ICA_STATE) -> Bus Creator/4  "ICABve_d_ICAState_convert"
  ICA_EPS/2(LKA_TRQ_FACT_REQ) -> Bus Creator/2  "OMAPve_g_Coefficient_toregulate_EPS_2"
  Bus Creator/1 -> Out1/1
  Demux/13 -> Subsystem1/24(stLCmode)  "[13]stLCMode"
  Demux/14 -> Subsystem1/25(stLFState)  "[14]stLFState"
  Demux/17 -> Subsystem1/28(stLCRmode_valid)  "[17]stLCRmode_valid"
  Demux/18 -> Subsystem1/29(stturn_lightState)  "[18]stturn_lightState"
  Demux/19 -> Subsystem1/30(stTLC_ALCmodeSW)  "[19]stTLC_ALCmodeSW"
  Demux/20 -> Subsystem1/31(stLC_SpdCndtFlg)  "[20]stLC_SpdCndtFlg"
  Bus Selector11/2 -> ICA_EPS/2(angle)  "<ICABve_g_SteerAngleCmd_convert>"
  Bus Selector11/4 -> ICA_EPS/4(torque)  "<ICABve_g_LKATorqueReq_Value_convert>"
  Subsystem1/9(TurnLightsCmd) -> Bus Creator1/9  "OMAPve_y_ADAS_TurnLightsCommand_2"
  Subsystem1/10(HWAActionSts) -> Bus Creator1/10  "OMAPve_y_ADAS_HWAActionSts_2"
  ICA_EPS/6(ICABve_d_LKATorqueReq_convert) -> Bus Creator/6  "ICABve_d_LKATorqueReq_convert"
  Subsystem1/7(stHWAmode) -> Bus Creator1/7  "OMAPve_y_ADAS_HWAMode_2"
  Subsystem1/8(LightControlValid) -> Bus Creator1/8  "OMAPve_y_ADAS_LightControlValid_2"
  Subsystem1/11(HWATurnOnIndicator) -> Bus Creator1/11  "OMAPve_y_ADAS_HWATurnOnIndicator_2"

== system OMAP/Runnable_OMAP_10ms_sys/OMAP_Module/Subsystem/EMS_Arbitration ==
  Input_ACCS : Inport
  Input_AEBS : Inport  Port=2
  Input_JABS : Inport  Port=3
  Input_FDMM : Inport  Port=4
  Input_IMAP : Inport  Port=5
  ACC/ICA_arb_AEB/JA : Subsystem
  Bus Selector3 : BusSelector  OutputSignals=FDMMve_d_JaFcnConf_convert
  FAPA_arb_ADAS : Subsystem
  Terminator3 : Terminator
  Arbitration_EMS : Outport
  wires:
  Bus Selector3/1 -> Terminator3/1  "<FDMMve_d_JaFcnConf_convert>"
  Input_FDMM/1 -> Bus Selector3/1
  Input_ACCS/1 -> ACC/ICA_arb_AEB/JA/1(Input_ACCS)
  Input_AEBS/1 -> ACC/ICA_arb_AEB/JA/2(Input_AEBS)
  Input_JABS/1 -> ACC/ICA_arb_AEB/JA/3(Input_JABS)
  Input_IMAP/1 -> FAPA_arb_ADAS/3(Input_FAPA), ACC/ICA_arb_AEB/JA/4(Input_IMAP)
  ACC/ICA_arb_AEB/JA/1(Out1) -> FAPA_arb_ADAS/1(Input_ACCICAAEBJA)
  ACC/ICA_arb_AEB/JA/2(Function_Acc_status) -> FAPA_arb_ADAS/2(Input_ACCstatus)
  FAPA_arb_ADAS/1(Arbitration_EMS) -> Arbitration_EMS/1

== system OMAP/Runnable_OMAP_10ms_sys/OMAP_Module/Subsystem/EPS_Default_Arbitration ==
  Input_AEBS : Inport
  Input_JABS : Inport  Port=2
  Input_LKAS : Inport  Port=3
  Input_ELKS : Inport  Port=4
  Input_ESAS : Inport  Port=5
  Input_ICA : Inport  Port=6
  Input_FDMM : Inport  Port=7
  Input_IMAP : Inport  Port=8
  AEB/JA_arb_ELK : Subsystem
  Bus Selector2 : BusSelector  OutputSignals=ESASve_y_ESA_State_convert
  FAPA_arb_ADAS : Subsystem
  ICA_arb_LKA : Subsystem
  LKA_arb_ELK : Subsystem
  Terminator2 : Terminator
  Arbitration_EPS : Outport
  wires:
  Input_FDMM/1 -> LKA_arb_ELK/1(Input_FDMM)
  Bus Selector2/1 -> Terminator2/1  "<ESASve_y_ESA_State_convert>"
  Input_ESAS/1 -> Bus Selector2/1
  Input_ICA/1 -> ICA_arb_LKA/1(Input_ICA)
  Input_LKAS/1 -> LKA_arb_ELK/2(Input_LKAS)
  LKA_arb_ELK/1(Out1) -> ICA_arb_LKA/2(Input_LKAELK)
  Input_AEBS/1 -> AEB/JA_arb_ELK/1(In1)
  Input_JABS/1 -> AEB/JA_arb_ELK/2(In2)
  Input_ELKS/1 -> AEB/JA_arb_ELK/3(In3)
  AEB/JA_arb_ELK/1(Out1) -> LKA_arb_ELK/3(Input_ELKS)
  ICA_arb_LKA/1(Out1) -> FAPA_arb_ADAS/1(Input_ICALKA)
  Input_IMAP/1 -> FAPA_arb_ADAS/2(Input_FAPA)
  FAPA_arb_ADAS/1(Arbitration_EPS) -> Arbitration_EPS/1

== system OMAP/Runnable_OMAP_10ms_sys/OMAP_Module/Subsystem/ESC_Arbitration ==
  Input_ACCS : Inport
  Input_AEBS : Inport  Port=2
  Input_JABS : Inport  Port=3
  Input_ELKS : Inport  Port=4
  Input_FDMM : Inport  Port=5
  Input_IMAP : Inport  Port=6
  ACC/ICA_arb_AEB/JA : Subsystem
  Bus Selector3 : BusSelector  OutputSignals=FDMMve_d_JaFcnConf_convert
  FAPA_arb_ADAS : Subsystem
  Terminator3 : Terminator
  Arbitration_ESC : Outport
  wires:
  Bus Selector3/1 -> Terminator3/1  "<FDMMve_d_JaFcnConf_convert>"
  Input_FDMM/1 -> Bus Selector3/1
  Input_ACCS/1 -> ACC/ICA_arb_AEB/JA/1(Input_ACCS)
  Input_AEBS/1 -> ACC/ICA_arb_AEB/JA/2(Input_AEBS)
  Input_JABS/1 -> ACC/ICA_arb_AEB/JA/3(Input_JABS)
  Input_IMAP/1 -> ACC/ICA_arb_AEB/JA/5(Input_IMAP), FAPA_arb_ADAS/3(Input_FAPA)
  Input_ELKS/1 -> ACC/ICA_arb_AEB/JA/4(Input_ELKS)
  ACC/ICA_arb_AEB/JA/1(Out1) -> FAPA_arb_ADAS/1(Input_ACCICAAEBJA1)
  ACC/ICA_arb_AEB/JA/2(Out2) -> FAPA_arb_ADAS/2(Input_ACCICAAEBJA2)
  FAPA_arb_ADAS/1(Arbitration_ESC) -> Arbitration_ESC/1

== system OMAP/Runnable_OMAP_10ms_sys/OMAP_Module/Subsystem/IC_Arbitration ==
  note: 仲裁内暂时将扭矩接口输出0，即ESA未参与仲裁逻辑，只支持ESA的单功能
  note: 仲裁#20——ICA与ACC
      | 1. ICA对仪表显示的独占信号，独立发送，不仲裁
      | 2. ACC对仪表显示的独占信号，独立发送，不仲裁
  note: 仲裁#2——ACC/ICA与FCW/JACW
      | 1. ACC/ICA算出的期望减速度>（标定值暂定-2.1）时，FCW强制不触发
      | 2. 否则，FCW/JACW根据自身的运算正常触发
  note: ACC与ICA强制转译
      | 关于文字提醒：
      | 当某一功能为开启 且 另一功能为关闭时，将关闭强制为0；其他情况按正常输出
  Input_ACCS : Inport
  Input_AEBS : Inport  Port=2
  Input_JABS : Inport  Port=3
  Input_LKAS : Inport  Port=4
  Input_ELKS : Inport  Port=5
  Input_ESAS : Inport  Port=6
  Input_ICA : Inport  Port=7
  Input_FDMM : Inport  Port=8
  Input_IMAP : Inport  Port=9
  ACC/ICA_arb_FCW/JACW : Subsystem
  ACC_ICA : Subsystem
  AEB/JA_arb_ELK : Subsystem
  AEB_arb_JA : Subsystem
  Bus Creator17 : BusCreator  Inputs=36
  Bus Selector : BusSelector  OutputSignals=OMAPve_y_LDW_Flag_2,OMAPve_y_LDW_Status_Display_2,OMAPve_y_LKA_Status_Display_2,OMAPve_y_LKA_action_indication_2,OMAPve_y_ADAS_ELKSts_2
  Bus Selector1 : BusSelector  OutputSignals=OMAPve_y_AEB_Alert_Req_2,OMAPve_y_AEB_Fault_Status_2,OMAPve_y_AEB_Switch_Status_2,OMAPve_y_AEB_tips_2,OMAPve_y_ADAS_JAFaultSt_2
  Bus Selector2 : BusSelector  OutputSignals=FDMMve_d_LkaFcnConf_convert
  Bus Selector3 : BusSelector  OutputSignals=HMI.OMAPve_y_ADAS_HWATurnOnIndicator_2,HMI.OMAPve_y_ADAS_HWAActionSts_2,HMI.OMAPve_y_ADAS_TurnLightsCommand_2,HMI.OMAPve_y_ADAS_LightControlValid_2,HMI.OMAPve_y_ADAS_HWAMode_2,HMI.OMAPve_y_TSR_Vision_Only_Sign_Type_2,HMI.OMAPve_y_ISA_Value_2,HMI.OMAPve_y_TJA_status_icon_2
  Bus Selector4 : BusSelector  OutputSignals=HMI.OMAPve_y_ACC_DesiredHeadway_Display_2,HMI.OMAPve_y_ACC_DesiredHeadway_Icon_Basic_2,HMI.OMAPve_y_ACC_Desired_Set_Speed_2,HMI.OMAPve_y_ACC_Set_Speed_Display_2,HMI.OMAPve_y_ACC_Vehicle_Icon_Display_2,HMI.OMAPve_y_RVVACC_Vehiclespeed_request_type_2,HMI.ACCSve_d_ACCMessagePrompt_convert,actuator.Deceleration_setpoint_device,HMI.OMAPve_y_ACC_HMI_TgtDisp_Flag_2,HMI.OMAPve_y_TARGET_POSITION_2,HMI.ACCSve_d_ACC_ISLCState_convert,HMI.ACCSve_d_ACC_ISLCDriverRemind_convert
  Bus Selector5 : BusSelector  OutputSignals=OMAPve_y_Hands_off_warning_2,OMAPve_y_HMI_Popup_Status_2,OMAPve_y_Vehicle_Lane_Display_2,OMAPve_y_ICA_HMI_Txt_Disp_2
  Bus Selector6 : BusSelector  OutputSignals=ELKSve_y_HMI_Popup_Status_convert
  Constant22 : Constant  Value=0  OutDataTypeStr=uint8
  Constant3 : Constant  Value=0  OutDataTypeStr=uint8
  Data Type Conversion{1..21,39,47..53,58..62} (34 alike) : DataTypeConversion  OutDataTypeStr=uint8
  ICA_arb_LKA/ELK : Subsystem
  LKA_arb_ELK : Subsystem
  Terminator1 : Terminator
  Terminator5 : Terminator
  Arbitration_IC : Outport
  wires:
  Input_ICA/1 -> ICA_arb_LKA/ELK/1(Input_ICA), Bus Selector3/1
  Input_ESAS/1 -> Terminator5/1
  Data Type Conversion17/1 -> Bus Creator17/15  "OMAPve_y_ACC_Pop_Up_Message_2"
  Data Type Conversion60/1 -> Bus Creator17/11  "OMAPve_y_ACC_Desired_Set_Speed_2"
  Data Type Conversion59/1 -> Bus Creator17/10  "OMAPve_y_ACC_DesiredHeadway_Icon_Basic_2"
  Data Type Conversion10/1 -> Bus Creator17/31  "OMAPve_y_LKA_Status_Display_2"
  Data Type Conversion13/1 -> Bus Creator17/35  "OMAPve_y_ICA_HMI_Txt_Disp_2"
  Data Type Conversion6/1 -> Bus Creator17/26  "OMAPve_y_HMI_Popup_Status_2"
  Data Type Conversion14/1 -> Bus Creator17/12  "OMAPve_y_ACC_Set_Speed_Display_2"
  Data Type Conversion58/1 -> Bus Creator17/9  "OMAPve_y_ACC_DesiredHeadway_Display_2"
  Data Type Conversion8/1 -> Bus Creator17/28  "OMAPve_y_LDW_Flag_2"
  Constant22/1 -> Bus Creator17/30  "OMAPve_y_LKA_Mode_from_Camera_2"
  Data Type Conversion16/1 -> Bus Creator17/14  "OMAPve_y_RVVACC_Vehiclespeed_request_type_2"
  Data Type Conversion11/1 -> Bus Creator17/33  "OMAPve_y_LKA_action_indication_2"
  Data Type Conversion12/1 -> Bus Creator17/36  "OMAPve_y_TJA_status_icon_2"
  Data Type Conversion18/1 -> Bus Creator17/21  "OMAPve_y_ACC_HMI_TgtDisp_Flag_2"
  Data Type Conversion5/1 -> Bus Creator17/25  "OMAPve_y_Hands_off_warning_2"
  Data Type Conversion7/1 -> Bus Creator17/27  "OMAPve_y_Vehicle_Lane_Display_2"
  Data Type Conversion19/1 -> Bus Creator17/22  "OMAPve_y_TARGET_POSITION_2"
  Data Type Conversion39/1 -> Bus Creator17/32  "OMAPve_y_LKA_Switch_State_2"
  Data Type Conversion9/1 -> Bus Creator17/29  "OMAPve_y_LDW_Status_Display_2"
  Data Type Conversion53/1 -> Bus Creator17/8  "OMAPve_y_TSR_Vision_Only_Sign_Type_2"
  Bus Creator17/1 -> Arbitration_IC/1  "Arbitration_IC"
  Data Type Conversion15/1 -> Bus Creator17/13  "OMAPve_y_ACC_Vehicle_Icon_Display_2"
  Data Type Conversion4/1 -> Bus Creator17/19  "OMAPve_y_AEB_tips_2"
  Data Type Conversion3/1 -> Bus Creator17/18  "OMAPve_y_AEB_Switch_Status_2"
  Data Type Conversion1/1 -> Bus Creator17/16  "OMAPve_y_AEB_Alert_Req_2"
  Data Type Conversion2/1 -> Bus Creator17/17  "OMAPve_y_AEB_Fault_Status_2"
  Bus Selector1/2 -> Data Type Conversion2/1  "<OMAPve_y_AEB_Fault_Status_2>"
  Bus Selector1/4 -> Data Type Conversion4/1  "<OMAPve_y_AEB_tips_2>"
  Bus Selector1/3 -> Data Type Conversion3/1  "<OMAPve_y_AEB_Switch_Status_2>"
  Input_LKAS/1 -> LKA_arb_ELK/2(Input_LKAS)
  Input_FDMM/1 -> LKA_arb_ELK/1(Input_FDMM), Bus Selector2/1
  Input_ACCS/1 -> Bus Selector4/1
  Bus Selector1/1 -> ACC/ICA_arb_FCW/JACW/2(<AEBSve_d_AEBAlertReq_convert>)  "<OMAPve_y_AEB_Alert_Req_2>"
  ACC/ICA_arb_FCW/JACW/1(Out1) -> Data Type Conversion1/1
  Bus Selector5/1 -> Data Type Conversion5/1  "<OMAPve_y_Hands_off_warning_2>"
  Bus Selector5/3 -> Data Type Conversion7/1  "<OMAPve_y_Vehicle_Lane_Display_2>"
  Bus Selector/1 -> Data Type Conversion8/1  "<OMAPve_y_LDW_Flag_2>"
  Bus Selector/2 -> Data Type Conversion9/1  "<OMAPve_y_LDW_Status_Display_2>"
  Bus Selector/3 -> Data Type Conversion10/1  "<OMAPve_y_LKA_Status_Display_2>"
  Bus Selector/4 -> Data Type Conversion11/1  "<OMAPve_y_LKA_action_indication_2>"
  Bus Selector2/1 -> Data Type Conversion39/1  "<FDMMve_d_LkaFcnConf_convert>"
  Input_ELKS/1 -> Bus Selector6/1, AEB/JA_arb_ELK/3(Input_ELKS)
  Input_JABS/1 -> AEB_arb_JA/2(Input_JABS), AEB/JA_arb_ELK/2(Input_JABS)
  Input_AEBS/1 -> AEB_arb_JA/1(Input_AEBS), AEB/JA_arb_ELK/1(Input_AEBS)
  AEB/JA_arb_ELK/1(Out1) -> LKA_arb_ELK/3(Input_ELKS)
  AEB_arb_JA/1(Out1) -> Bus Selector1/1
  Bus Selector3/6 -> Data Type Conversion53/1  "<OMAPve_y_TSR_Vision_Only_Sign_Type_2>"
  Bus Selector3/7 -> ?  "<OMAPve_y_ISA_Value_2>"
  Bus Selector3/8 -> Data Type Conversion12/1  "<OMAPve_y_TJA_status_icon_2>"
  Bus Selector4/1 -> Data Type Conversion58/1  "<OMAPve_y_ACC_DesiredHeadway_Display_2>"
  Bus Selector4/2 -> Data Type Conversion59/1  "<OMAPve_y_ACC_DesiredHeadway_Icon_Basic_2>"
  Bus Selector4/3 -> Data Type Conversion60/1  "<OMAPve_y_ACC_Desired_Set_Speed_2>"
  Bus Selector4/4 -> Data Type Conversion14/1  "<OMAPve_y_ACC_Set_Speed_Display_2>"
  Bus Selector4/5 -> Data Type Conversion15/1  "<OMAPve_y_ACC_Vehicle_Icon_Display_2>"
  Bus Selector4/6 -> Data Type Conversion16/1  "<OMAPve_y_RVVACC_Vehiclespeed_request_type_2>"
  Bus Selector4/7 -> ACC_ICA/1(ACC_Message)  "<ACCSve_d_ACCMessagePrompt_convert>"
  Bus Selector4/8 -> ACC/ICA_arb_FCW/JACW/1(Input_ACCS)  "<Deceleration_setpoint_device>"
  Bus Selector4/9 -> Data Type Conversion18/1  "<OMAPve_y_ACC_HMI_TgtDisp_Flag_2>"
  Bus Selector4/10 -> Data Type Conversion19/1  "<OMAPve_y_TARGET_POSITION_2>"
  LKA_arb_ELK/1(Out1) -> ICA_arb_LKA/ELK/2(Input_LKAELK), Bus Selector/1
  ICA_arb_LKA/ELK/1(Out1) -> Bus Selector5/1
  Data Type Conversion20/1 -> Bus Creator17/34  "OMAPve_y_ADAS_ELKSts_2"
  Bus Selector/5 -> Data Type Conversion20/1  "<OMAPve_y_ADAS_ELKSts_2>"
  Input_IMAP/1 -> Terminator1/1
  Bus Selector5/2 -> Data Type Conversion6/1  "<OMAPve_y_HMI_Popup_Status_2>"
  Bus Selector5/4 -> ACC_ICA/2(ICA_Message)  "<OMAPve_y_ICA_HMI_Txt_Disp_2>"
  Data Type Conversion47/1 -> Bus Creator17/20  "OMAPve_y_ADAS_JAFaultSt_2"
  Bus Selector1/5 -> Data Type Conversion47/1  "<OMAPve_y_ADAS_JAFaultSt_2>"
  Data Type Conversion48/1 -> Bus Creator17/5  "OMAPve_y_ADAS_TurnLightsCommand_2"
  Bus Selector3/3 -> Data Type Conversion48/1  "<OMAPve_y_ADAS_TurnLightsCommand_2>"
  Bus Selector4/11 -> Data Type Conversion49/1  "<ACCSve_d_ACC_ISLCState_convert>"
  Bus Selector4/12 -> Data Type Conversion50/1  "<ACCSve_d_ACC_ISLCDriverRemind_convert>"
  Data Type Conversion49/1 -> Bus Creator17/23  "OMAPve_y_ADAS_ISLCState_2"
  Data Type Conversion50/1 -> Bus Creator17/24  "OMAPve_y_ADAS_ISLCDriverRemind_2"
  Data Type Conversion51/1 -> Bus Creator17/6  "OMAPve_y_ADAS_LightControlValid_2"
  Data Type Conversion52/1 -> Bus Creator17/7  "OMAPve_y_ADAS_HWAMode_2"
  Bus Selector3/4 -> Data Type Conversion51/1  "<OMAPve_y_ADAS_LightControlValid_2>"
  Bus Selector3/5 -> Data Type Conversion52/1  "<OMAPve_y_ADAS_HWAMode_2>"
  Data Type Conversion61/1 -> Bus Creator17/4  "OMAPve_y_ADAS_HWAActionSts_2"
  Data Type Conversion62/1 -> Bus Creator17/3  "OMAPve_y_ADAS_HWATurnOnIndicator_2"
  Bus Selector3/2 -> Data Type Conversion61/1  "<OMAPve_y_ADAS_HWAActionSts_2>"
  Bus Selector3/1 -> Data Type Conversion62/1  "<OMAPve_y_ADAS_HWATurnOnIndicator_2>"
  Constant3/1 -> Bus Creator17/2  "OMAPve_y_ADAS_ESAFaultSt_2"
  Data Type Conversion21/1 -> Bus Creator17/1  "OMAPve_y_ADAS_ELKPopupMessage_2"
  Bus Selector6/1 -> Data Type Conversion21/1  "<ELKSve_y_HMI_Popup_Status_convert>"
  ACC_ICA/1(ACC_Message_out) -> Data Type Conversion17/1
  ACC_ICA/2(ICA_Message_out) -> Data Type Conversion13/1

== system OMAP/Runnable_OMAP_10ms_sys/OMAP_Module/ACCS_Direct/ACCS_Define/ACC_State_Synthesis(ACC_SS) ==
  Input_ACCS : Inport
  Bus Selector : BusSelector  OutputSignals=Deceleration_setpoint_device,TminDownGear,TminUpGear,StAcvTqWhlPTPotReq,PotACCTqReq,Function_Acc_status,ACCTqReq,Powertrain_torquewheel_request,TYPE_RAPPORT,MDD_Decelerationcontrol_request,MDD_deceleration_type,Power_steering_power_cut3F2
  Bus Selector2 : BusSelector  OutputSignals=ACCSve_d_ACC_State_convert
  Compare To Constant1 : simulink/Logic and Bit Operations/Compare To Constant  relop===  const=0  OutDataTypeStr=boolean
  Compare To Constant2 : simulink/Logic and Bit Operations/Compare To Constant  relop===  const=1  OutDataTypeStr=boolean
  Compare To Constant5 : simulink/Logic and Bit Operations/Compare To Constant  relop===  const=2  OutDataTypeStr=boolean
  Compare To Constant6 : simulink/Logic and Bit Operations/Compare To Constant  relop===  const=3  OutDataTypeStr=boolean
  Compare To Constant7 : simulink/Logic and Bit Operations/Compare To Constant  relop===  const=15  OutDataTypeStr=boolean
  If Action Subsystem2 : Subsystem  TreatAsAtomicUnit=on
  If Action Subsystem3 : Subsystem  TreatAsAtomicUnit=on
  If1 : If  IfExpression=u1 == 1
  Logical Operator1 : Logic  Operator=OR  Inputs=5  AllPortsSameDT=off  OutDataTypeStr=boolean
  Merge : Merge
  ACC_Control_Signal : Outport
  tag scope: ob_ACC_ACCTqReq=global, ob_ACC_Deceleration_setpoint_device=global, ob_ACC_Function_Acc_status=global, ob_ACC_MDD_Decelerationcontrol_request=global, ob_ACC_MDD_deceleration_type=global, ob_ACC_PotACCTqReq=global, ob_ACC_Power_steering_power_cut3F2=global, ob_ACC_Powertrain_torquewheel_request=global, ob_ACC_StAcvTqWhlPTPotReq=global, ob_ACC_TYPE_RAPPORT=global, ob_ACC_TminDownGear=global, ob_ACC_TminUpGear=global
  wires:
  Input_ACCS/1 -> Bus Selector2/1, If Action Subsystem3/1(ACT_Control_Signal)
  Bus Selector/12 -> [ob_ACC_Power_steering_power_cut3F2]  "<Power_steering_power_cut3F2>"
  Bus Selector/11 -> [ob_ACC_MDD_deceleration_type]  "<MDD_deceleration_type>"
  Bus Selector/10 -> [ob_ACC_MDD_Decelerationcontrol_request]  "<MDD_Decelerationcontrol_request>"
  Bus Selector/9 -> [ob_ACC_TYPE_RAPPORT]  "<TYPE_RAPPORT>"
  Bus Selector/8 -> [ob_ACC_Powertrain_torquewheel_request]  "<Powertrain_torquewheel_request>"
  Bus Selector/7 -> [ob_ACC_ACCTqReq]  "<ACCTqReq>"
  Bus Selector/6 -> [ob_ACC_Function_Acc_status]  "<Function_Acc_status>"
  Bus Selector/5 -> [ob_ACC_PotACCTqReq]  "<PotACCTqReq>"
  Bus Selector/4 -> [ob_ACC_StAcvTqWhlPTPotReq]  "<StAcvTqWhlPTPotReq>"
  Bus Selector/3 -> [ob_ACC_TminUpGear]  "<TminUpGear>"
  Bus Selector/2 -> [ob_ACC_TminDownGear]  "<TminDownGear>"
  Bus Selector/1 -> [ob_ACC_Deceleration_setpoint_device]  "<Deceleration_setpoint_device>"
  Merge/1 -> ACC_Control_Signal/1, Bus Selector/1  "Control_Ouput"
  If Action Subsystem3/1(Control_Ouput) -> Merge/2
  If Action Subsystem2/1(Control_Ouput) -> Merge/1
  If1/2 -> If Action Subsystem3/Action
  If1/1 -> If Action Subsystem2/Action
  Logical Operator1/1 -> If1/1
  Compare To Constant7/1 -> Logical Operator1/5
  Compare To Constant6/1 -> Logical Operator1/4
  Compare To Constant5/1 -> Logical Operator1/3
  Compare To Constant1/1 -> Logical Operator1/1
  Compare To Constant2/1 -> Logical Operator1/2
  Bus Selector2/1 -> Compare To Constant1/1, Compare To Constant2/1, Compare To Constant5/1, Compare To Constant6/1, Compare To Constant7/1, If Action Subsystem2/1(In1)  "<ACCSve_d_ACC_State_convert>"
